simulink model "Non_linear_model"  (R2025a)
settings: Solver=VariableStepAuto  StartTime=0.0  StopTime=10  RelTol=1e-3
model workspace: external: MATLAB File C:\Users\josep\Documents\mecatro_mines_05\matlab\linear_model_constants.m (data not in the file)
values from neighbouring files (symbols this model uses):
  A_W = [0 1 0 ... (first row only)    [linear_model_constants.m]
  B_W = [-d_i 0 ... (first row only)    [linear_model_constants.m]
  C_W = [2/rho 0 -2]    [linear_model_constants.m]
  d = 0.058    [linear_model_constants.m]
  d_i = 0.0915    [linear_model_constants.m]
  g = 9.81    [linear_model_constants.m]
  Itot_y = I_y + 2 * Iw_y    (= 0.00916366)    [linear_model_constants.m]
  Iw_y = 2.5233 * 1e-4    (= 0.00025233)    [linear_model_constants.m]
  k = 0.3346    [linear_model_constants.m]
  L = place(A_W', C_W', p_L)'    [linear_model_constants.m]
  M = m_b + 2 * m_w    (= 1.266)    [linear_model_constants.m]
  m_b = 1.206    [linear_model_constants.m]
  N = [alpha_ 0 beta_ 0 ... (first row only)    [linear_model_constants.m]
  R = 2.181818    [linear_model_constants.m]
  rho = 0.050    (= 0.05)    [linear_model_constants.m]
libraries: simulink x1
settings Model: Creator=josep  LastModifiedBy=josep

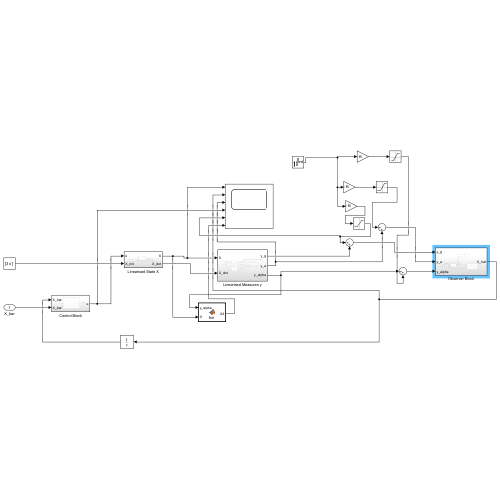
[thumbnail: Simulink's stored preview of the top-level diagram]
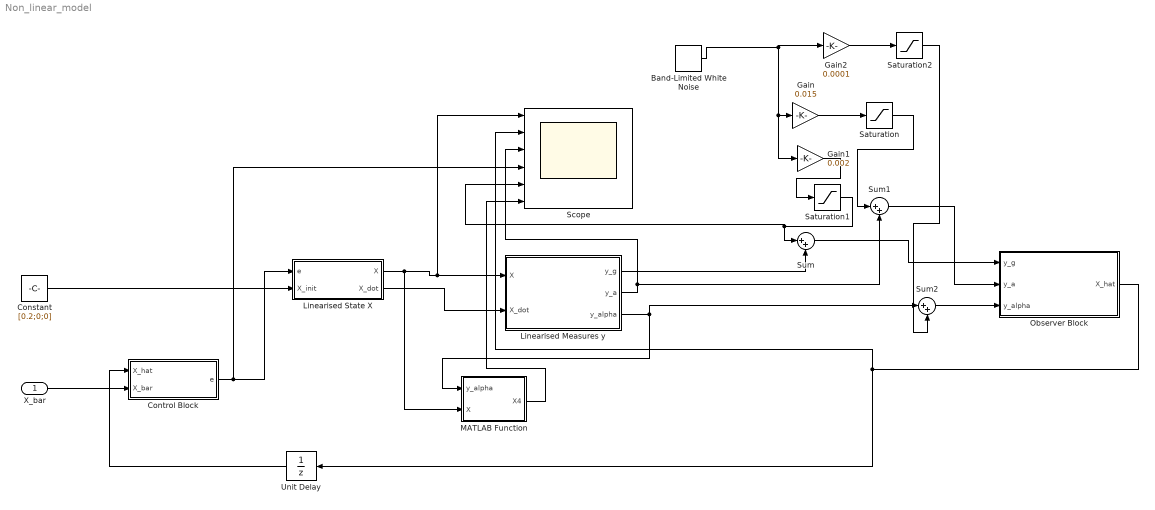
== system Non_linear_model ==
  X_bar : Inport
  Band-Limited White Noise : simulink/Sources/Band-Limited White Noise  Cov=[0.1]  Ts=0.1  seed=[23341]
  Constant : Constant  Value=[0.2;0;0]
  Control Block : Subsystem
  Gain : Gain  Gain=0.015
  Gain1 : Gain  Gain=0.002
  Gain2 : Gain  Gain=0.0001
  Linearised Measures y : Subsystem
  Linearised State X : Subsystem
  MATLAB Function : MATLAB Function  TreatAsAtomicUnit=on
  Observer Block : Subsystem
  Saturation : Saturate  UpperLimit=0.015  LowerLimit=-0.015
  Saturation1 : Saturate  UpperLimit=0.002  LowerLimit=-0.002
  Saturation2 : Saturate  UpperLimit=0.015  LowerLimit=-0.015
  Scope : Scope  NumInputPorts=6
      settings: ActiveDisplayYMinimum=-2.6750581044154509  ActiveDisplayYMaximum=3.5501509335258414
  Sum : Sum  Inputs=|++
  Sum1 : Sum  Inputs=|++
  Sum2 : Sum  Inputs=|++
  Unit Delay : UnitDelay  SampleTime=0.01  HasFrameUpgradeWarning=on
  wires:
  Linearised State X/1(X) -> MATLAB Function/2(X), Scope/1, Linearised Measures y/1(X)
  Linearised Measures y/1(y_g) -> Sum/2
  Linearised Measures y/2(y_a) -> Scope/3, Sum1/2
  X_bar/1 -> Control Block/2(X_bar)
  Linearised State X/2(X_dot) -> Linearised Measures y/2(X_dot)
  Constant/1 -> Linearised State X/2(X_init)
  Observer Block/1(X_hat) -> Unit Delay/1, Scope/2
  Control Block/1(e) -> Scope/4, Linearised State X/1(e)
  MATLAB Function/1(X4) -> Scope/6
  Unit Delay/1 -> Control Block/1(X_hat)
  Linearised Measures y/3(y_alpha) -> Sum2/1, MATLAB Function/1(y_alpha)
  Sum/1 -> Observer Block/1(y_g)
  Sum1/1 -> Observer Block/2(y_a)
  Saturation/1 -> Sum1/1
  Saturation1/1 -> Scope/5, Sum/1
  Gain/1 -> Saturation/1
  Band-Limited White Noise/1 -> Gain2/1, Gain/1, Gain1/1
  Gain1/1 -> Saturation1/1
  Gain2/1 -> Saturation2/1
  Saturation2/1 -> Sum2/2
  Sum2/1 -> Observer Block/3(y_alpha)

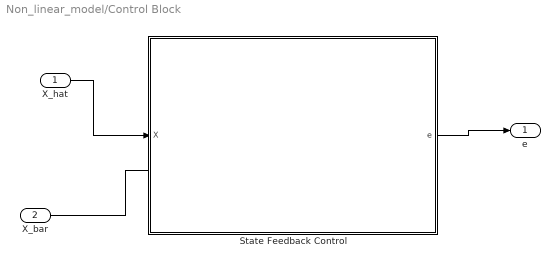
== system Non_linear_model/Control Block ==
  X_hat : Inport
  X_bar : Inport  Port=2
  State Feedback Control : MATLAB Function  TreatAsAtomicUnit=on
  e : Outport
  wires:
  X_hat/1 -> State Feedback Control/1(X)
  X_bar/1 -> ?
  State Feedback Control/1(e) -> e/1

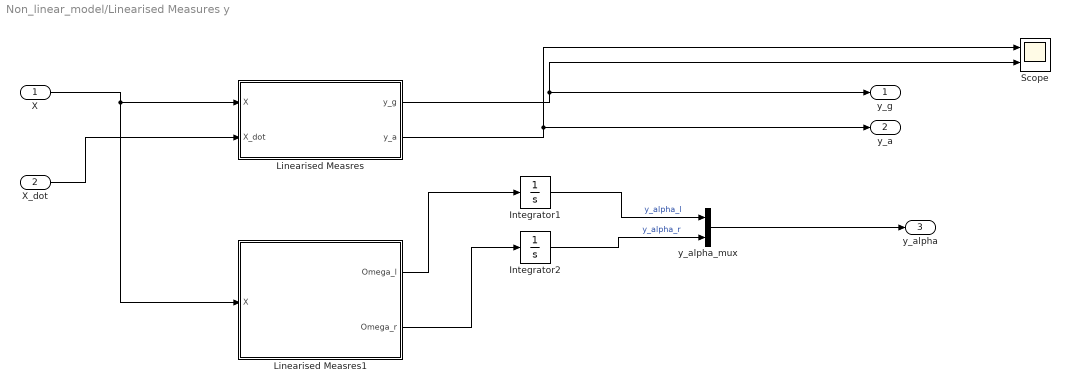
== system Non_linear_model/Linearised Measures y ==
  X : Inport
  X_dot : Inport  Port=2
  Integrator1 : Integrator
  Integrator2 : Integrator
  Linearised Measres : MATLAB Function  TreatAsAtomicUnit=on
  Linearised Measres1 : MATLAB Function  TreatAsAtomicUnit=on
  Scope : Scope  NumInputPorts=2
      settings: ActiveDisplayYMinimum=-0.51043745646463368  ActiveDisplayYMaximum=1.2338081847305338  DataLoggingVariableName=ScopeData2
  y_alpha_mux : Mux  Inputs=2
  y_g : Outport  PortDimensions=3
  y_a : Outport  Port=2
  y_alpha : Outport  Port=3
  wires:
  X/1 -> Linearised Measres1/1(X), Linearised Measres/1(X)
  Linearised Measres/2(y_a) -> y_a/1, Scope/1
  Linearised Measres/1(y_g) -> y_g/1, Scope/2
  y_alpha_mux/1 -> y_alpha/1
  Linearised Measres1/1(Omega_l) -> Integrator1/1
  Integrator1/1 -> y_alpha_mux/1  "y_alpha_l"
  Linearised Measres1/2(Omega_r) -> Integrator2/1
  Integrator2/1 -> y_alpha_mux/2  "y_alpha_r"
  X_dot/1 -> Linearised Measres/2(X_dot)

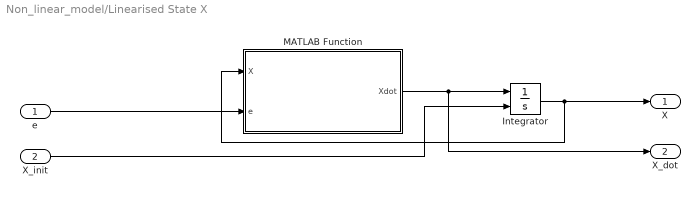
== system Non_linear_model/Linearised State X ==
  e : Inport  PortDimensions=2
  X_init : Inport  Port=2  PortDimensions=3
  Integrator : Integrator  InitialConditionSource=external
  MATLAB Function : MATLAB Function  TreatAsAtomicUnit=on
  X : Outport  PortDimensions=3
  X_dot : Outport  Port=2  PortDimensions=3
  wires:
  e/1 -> MATLAB Function/2(e)
  MATLAB Function/1(Xdot) -> X_dot/1, Integrator/1
  Integrator/1 -> MATLAB Function/1(X), X/1
  X_init/1 -> Integrator/2

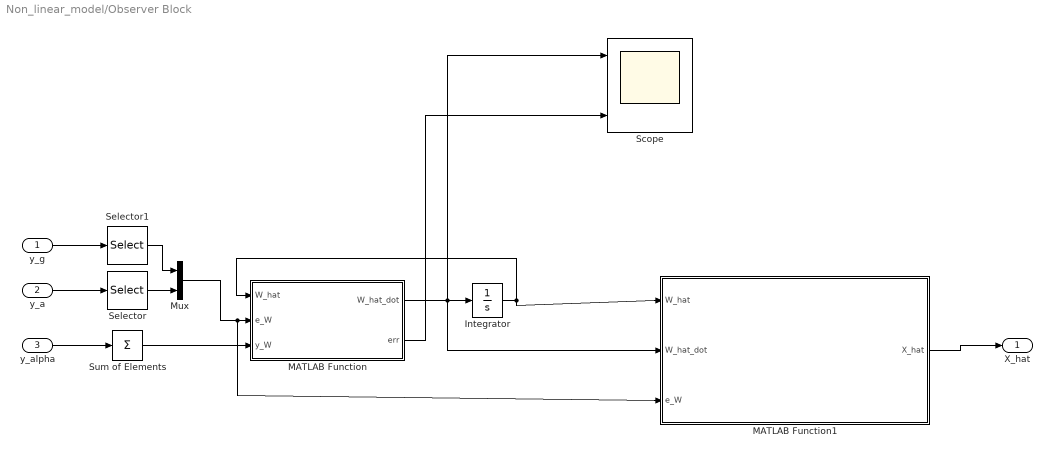
== system Non_linear_model/Observer Block ==
  y_g : Inport  PortDimensions=3
  y_a : Inport  Port=2
  y_alpha : Inport  Port=3  PortDimensions=2
  Integrator : Integrator  InitialCondition=[0; 0; 0]
  MATLAB Function : MATLAB Function  TreatAsAtomicUnit=on
  MATLAB Function1 : MATLAB Function  TreatAsAtomicUnit=on
  Mux : Mux  Inputs=2
  Scope : Scope  NumInputPorts=3
      settings: ActiveDisplayYMinimum=-0.0067554823375903985  ActiveDisplayYMaximum=0.01622805881894273
  Selector : Selector  InputPortWidth=3  IndexOptions=Index vector (dialog)  Indices=1  OutputSizes=1
  Selector1 : Selector  InputPortWidth=3  IndexOptions=Index vector (dialog)  Indices=2  OutputSizes=1
  Sum of Elements : Sum  Inputs=+
  X_hat : Outport  PortDimensions=4
  wires:
  MATLAB Function/1(W_hat_dot) -> MATLAB Function1/2(W_hat_dot), Integrator/1, Scope/1
  Integrator/1 -> MATLAB Function/1(W_hat), MATLAB Function1/1(W_hat)
  MATLAB Function1/1(X_hat) -> X_hat/1
  y_a/1 -> Selector/1
  y_g/1 -> Selector1/1
  y_alpha/1 -> Sum of Elements/1
  Selector1/1 -> Mux/1
  Selector/1 -> Mux/2
  Mux/1 -> MATLAB Function1/3(e_W), MATLAB Function/2(e_W)
  Sum of Elements/1 -> MATLAB Function/3(y_W)
  MATLAB Function/2(err) -> Scope/3

== matlab function Non_linear_model/Linearised Measures y/Linearised Measres ==
  data: X input; y_g output; y_a output; X_dot input; g parameter; d_i parameter
function [y_g, y_a] = lin_y(X, X_dot, g, d_i)

% y_g is the 3 dimensional output that is given by C_1 X + b_1
% y_a is the 3 dimensional output, that is given by C_2 X + b_2

theta     = X(1);
theta_dot = X(3);
u_dot      = X_dot(2);


% Gyroscope (body angular rates)
y_g = [0;
      theta_dot;
      0];

% Accelerometer (specific acceleration in IMU frame)
y_a = [u_dot * cos(theta) - g * sin(theta) + d_i*X_dot(3);
      0;
      u_dot * sin(theta) + g * cos(theta) - d_i*theta_dot^2];

== matlab function Non_linear_model/Linearised State X/MATLAB Function ==
  data: X input; Xdot output; e input; rho parameter; R parameter; k parameter; M parameter; m_b parameter; Iw_y parameter; d parameter; Itot_y parameter; g parameter
function Xdot = nonlinmodel(X, e, rho, R, k, M, m_b, Iw_y, d, Itot_y, g)

theta     = X(1);
u         = X(2);

theta_dot = X(3);

Ul = e(1);
Ur = e(2);



omega = u / rho - theta_dot;

il = Ul/R - (k/R) * omega;
ir = Ur/R - (k/R) * omega;

tau_l = k * il;
tau_r = k * ir;




A11 = M + 2*Iw_y/rho^2;
A12 = m_b*d * cos(theta);
A21 = m_b*d * cos(theta);
A22 = Itot_y + m_b*d^2;

B1 = (1/rho)*(tau_l + tau_r) + m_b*d*sin(theta)*theta_dot^2;
B2 = -(tau_l + tau_r) + m_b*d*g*sin(theta);

A_ = [A11, A12;
      A21, A22];

B_ = [B1;
      B2];
sol = A_\B_;

u_dot       = sol(1);
theta_ddot  = sol(2);

Xdot = zeros(3,1);
Xdot(1) = theta_dot;
Xdot(2) = u_dot;
Xdot(3) = theta_ddot;
end

== matlab function Non_linear_model/Linearised Measures y/Linearised Measres1 ==
  data: X input; Omega_l output; Omega_r output; rho parameter
function [Omega_l, Omega_r] = lin_Omega(X, rho)
theta_dot = X(3);
u=X(2);
Omega_l_r = (1/rho)*u-theta_dot;
Omega_l = Omega_l_r;
Omega_r = Omega_l_r;

== matlab function Non_linear_model/Observer Block/MATLAB Function ==
  data: W_hat input; e_W input; y_W input; W_hat_dot output size=3; A_W parameter; C_W parameter; B_W parameter; L parameter; err output
function [W_hat_dot, err] = observer(W_hat, e_W, y_W, A_W, C_W, B_W, L)

% Write the observer equation out, W_hat_dot = A * W_hat + B * e + L (y -
% y_hat) where e is a 2d vector as a linear combination of y_g and y_a




y_hat = C_W * W_hat;

err = y_W - y_hat;
W_hat_dot = A_W * W_hat + B_W * e_W + (y_W - y_hat) * L;

== matlab function Non_linear_model/Observer Block/MATLAB Function1 ==
  data: W_hat input; X_hat output; W_hat_dot input; e_W input; d_i parameter; N parameter
function X_hat = W_hat_to_X_hat(W_hat, W_hat_dot, e_W, d_i, N)

p = W_hat(1);
theta = W_hat(3);
theta_dot = e_W(1);
u = W_hat(2) - d_i * theta_dot;

X_hat = N * [p; u; theta; theta_dot];

== matlab function Non_linear_model/Control Block/State Feedback Control ==
  data: X input; e output; K parameter
function e = state_feedback(X, K)
    % Function that gives the control signal for the eqn
    % X_dot = (A - BK)X + Bkr, where u = -KX + r, where r is
    % a reference consant (or non constant maybe ?)
    
    % solving the system, we get that equilibrium will be reached at x_bar =
    % - (A - BK)^-1 Br, which means that if we set a reference r, we can control
    % where the system stabilises to. Thus, r = (K - B^-1 A)x_bar
    
    % the control signal "u" here is given by the sum of components of e, so e
    % should be 
    
      e_unlimited = - K * X;
      e = [min(max(e_unlimited(1), -12), 12)
           min(max(e_unlimited(2), -12), 12)];
end

== matlab function Non_linear_model/MATLAB Function ==
  data: y_alpha input; X4 output; X input; rho parameter
function X4 = fcn(y_alpha , X, rho)

X4 = [((y_alpha(1)+y_alpha(2))/2+X(1))*rho; X(2) ; X(1) ; X(3)];
